simulink model "SDS_CBC_forcopyandpaste"  (R2018b)
settings: Solver=VariableStepAuto  StartTime=0.0  StopTime=10.0  RelTol=1e-3
PostLoadFcn:
  | , if any(exist('dsrtsu_mdlpostloadfcn', 'file') == [2, 3, 6]), try dsrtsu_mdlpostloadfcn('Execute', bdroot); catch fprintf('Error in PostLoadFcn (dsrtsu_mdlpostloadfcn) for model "%s":\n %s\n', bdroot, lasterr); end, end,
libraries: rtican x2, simulink x1
settings Model: DSRTSU_INTERNAL_RTI_VER=520  DSRTSU_INTERNAL_RTI_TYPE=rti1401  Creator=cordunoalbarran  LastModifiedBy=cordunoalbarran

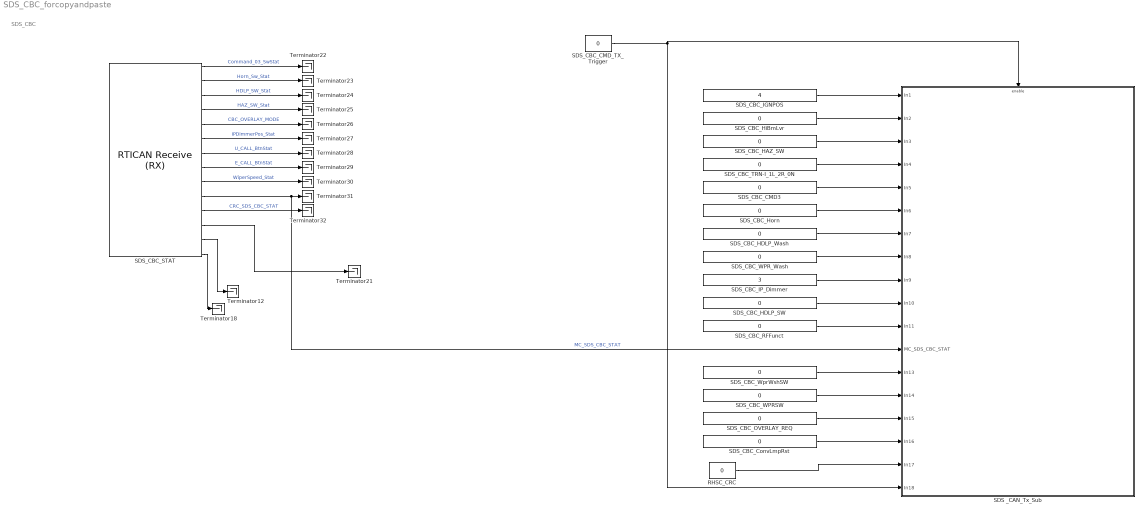
== system SDS_CBC_forcopyandpaste ==
  note: SDS_CBC
  RHSC_CRC : Constant  Value=0  OutDataTypeStr=Inherit: Inherit via back propagation
  "SDS _CAN_Tx_Sub " : Subsystem
  SDS_CBC_CMD3 : Constant  Value=0
  SDS_CBC_CMD_TX_Trigger : Constant  Value=0  OutDataTypeStr=Inherit: Inherit via back propagation
  SDS_CBC_ConvLmpRst : Constant  Value=0
  SDS_CBC_HAZ_SW : Constant  Value=0
  SDS_CBC_HDLP_SW : Constant  Value=0
  SDS_CBC_HDLP_Wash : Constant  Value=0
  SDS_CBC_HiBmLvr : Constant  Value=0
  SDS_CBC_Horn : Constant  Value=0
  SDS_CBC_IGNPOS : Constant  Value=4  OutMin=0  OutMax=6
  SDS_CBC_IP_Dimmer : Constant  Value=3
  SDS_CBC_OVERLAY_REQ : Constant  Value=0
  SDS_CBC_RFFunct : Constant  Value=0
  SDS_CBC_STAT : rtican/RTICAN Receive (RX)   Reserved1=[]  Reserved2=[]  Reserved3=[]  Reserved4=[]  SfcnMessage=[]  Msg_Struct=[]  BoardTypeNo=[]  BoardNo=[]  ChannelNo=[]  Parameters=[]  DialogFcn=[]  UnitName=[]  Revision=[]  UnitValues=[]  DSProperties=struct('RTI',struct('Version',uint32(5),'BlockType',struct('isSLSource',uint8(1),'isSLSink',uint8(1),'isHWSource',uint8(0),'isHWSink',uint8(0),'isSetup',uint8(0),'isInline',uint8(1),'isNonInline',uint8(0),'isInterrupt',uint8(0),'isChannelwise',uint8(0)),'IOBoardType','RTICAN','UnitType','MESSAGE','Identifier','RX','DialogType','MSVC','BlockSet','RTICAN','SlaveProcessor','CAN'))  RTIBlockInterface=struct('OutputPortsWidth',int32([1 1 1 1 1 1 1 1 1 1 1 1 1 1]),'OutputPortsActive',ones(1,14),'OutputPortsName',{{'Command_03_SwStat','Horn_Sw_Stat','HDLP_SW_Stat','HAZ_SW_Stat','CBC_OVERLAY_MODE','IPDimmerPos_Stat','U_CALL_BtnStat','E_CALL_BtnStat','WiperSpeed_Stat','MC_SDS_CBC_STAT','CRC_SDS_CBC_STAT',['RX status'],['RX time'],['RX delta time']}},'OutputPortsDataType',{{'SS_UINT8','SS_BOOLEAN','SS_UINT8','SS_BOOLEAN','SS_UINT8','SS_UINT8','SS_UINT8','SS_UINT8','SS_UINT8','SS_UINT8','SS_UINT8','SS_DOUBLE','SS_DOUBLE','SS_DOUBLE'}},'OutputPortsLabel',{{'Command_03_SwStat','Horn_Sw_Stat','HDLP_SW_Stat','HAZ_SW_Stat','CBC_OVERLAY_MODE','IPDimmerPos_Stat','U_CALL_BtnStat','E_CALL_BtnStat','WiperSpeed_Stat','MC_SDS_CBC_STAT','CRC_SDS_CBC_STAT','','',''}},'OutputPortsLabelMode','ON','InputPortsWidth',int32(0),'InputPortsActive',0,'DialogFcn','rtican_message_interface_gui','BlockDisplay',{{'','center'}},'IconTransparency','on','ParameterTunableNames',{{}},'InitLevel',3,'BlockName',struct('Token',{{'SDS_CBC_STAT'}}),'SampleTime',{{-1}},'TriggerPort',{{'none'}},'EnablePort',{{'none'}})  RTIBlockParameters=struct('BoardTypeNo',{{1,'OFF',[]}},'BoardNo',{{1,'ON',[1 16]}},'ChannelNo',{{1,'ON',[1 2]}},'Parameters',{{struct('DataFileSupport',struct('DataFileSelectedMaster',1,'DataFileSelectedLocal',1,'DataFileName',['c:\intrepidcs\pacifica dbc\e4a_r4_ccan_cr11690_mod.dbc|'],'DataFileDate',{{{['26-Feb-2019 09:25:05']}}},'SelectedFile',['..\..\..\..\..\..\..\intrepidcs\pacifica dbc\e4a_r4_ccan_cr11690_mod.dbc'],'InterfaceFcn','rtican_dbc_file_parser'),'Options',struct('StatusSelected',1,'TimeSelected',1,'DeltaTimeSelected',1,'BytePortSelected',0,'MessageLengthSelected',0,'TriggerPort',struct('Selected',0,'TriggerType',0),'UserCoding',struct('Selected',0,'InterfaceFile','UserDecodingFile','FcnName','UserDecodeFcn','InportSelected',0,'InportWidth',1,'OutportSelected',0,'OutportWidth',1),'EnablePortSelected',0,'SignalOnPortnameSelected',1,'UseRXService',0),'Message',struct('MsgOnBlocknameSelected',1,'MsgName','SDS_CBC_STAT','MsgIdFormat',0,'MsgId',858,'MsgLength',5,'NumSignals',11,'SampleTime',-1,'Signal',struct('SgnName',{'Command_03_SwStat','Horn_Sw_Stat','HDLP_SW_Stat','HAZ_SW_Stat','CBC_OVERLAY_MODE','IPDimmerPos_Stat','U_CALL_BtnStat','E_CALL_BtnStat','WiperSpeed_Stat','MC_SDS_CBC_STAT','CRC_SDS_CBC_STAT'},'SgnStartBit',{0,2,4,7,13,16,20,22,24,28,32},'SgnLength',{2,1,3,1,3,4,2,2,2,4,8},'SgnType',{0,0,0,0,0,0,0,0,0,0,0},'ModeValue',{-1,-1,-1,-1,-1,-1,-1,-1,-1,-1,-1},'DataType',{0,0,0,0,0,0,0,0,0,0,0},'ByteLayout',{0,0,0,0,0,0,0,0,0,0,0},'Factor',{1,1,1,1,1,1,1,1,1,1,1},'Offset',{0,0,0,0,0,0,0,0,0,0,0},'SgnComment',{{['Steering wheel switch 3 - Actual Switch Status (mode button)']},{['Physical Horn Pad Status']},{['Headlamp switch actual status']},{['Hazard Switch Actual Status; Not Pressed = [0], Pressed = [1];']},{['CBC Overlay Mode']},{['IP Dimmer Position Status to RHSC2']},{['Ucall button status to RHSC2']},{['Ecall button status to RHSC2']},{['Speed of wiper from RLS']},{['Message counter']},{['CRC-checksum byte 1 to 4 according to SAE J1850']}},'SgnUnit',{'','','','','','','','','','',''},'Min',{0,0,0,0,0,0,0,0,0,0,0},'Max',{0,0,0,0,0,0,0,0,0,15,0},'SLDataType',{'SS_UINT8','SS_BOOLEAN','SS_UINT8','SS_BOOLEAN','SS_UINT8','SS_UINT8','SS_UINT8','SS_UINT8','SS_UINT8','SS_UINT8','SS_UINT8'}),'MsgIdNumFormat',0,'MsgComment',{{''}}),'Version',1.2,'general',struct('isFromLib',0)),'OFF',[]}},'GroupId',{{struct('Group',{{'RTICAN'}},'No',1,'Behavior',{{'NAMECHANGE'}},'BlockType',{{'SINK'}},'NameChangeFlag',0),'OFF',[]}},'SFcnRTICANMessage',{{struct('MsgType','RX','SFcnPortType','Scalar','MsgName','SDS_CBC_STAT','MsgIdFormat','STD','MsgId',858,'MsgLength',5,'NumSignals',11,'SampleTime',-1,'Signal',struct('SgnName',{'Command_03_SwStat','Horn_Sw_Stat','HDLP_SW_Stat','HAZ_SW_Stat','CBC_OVERLAY_MODE','IPDimmerPos_Stat','U_CALL_BtnStat','E_CALL_BtnStat','WiperSpeed_Stat','MC_SDS_CBC_STAT','CRC_SDS_CBC_STAT'},'SgnStartBit',{0,2,4,7,13,16,20,22,24,28,32},'SgnLength',{2,1,3,1,3,4,2,2,2,4,8},'SgnType',{'standard','standard','standard','standard','standard','standard','standard','standard','standard','standard','standard'},'ModeValue',{-1,-1,-1,-1,-1,-1,-1,-1,-1,-1,-1},'DataType',{['unsigned int'],['unsigned int'],['unsigned int'],['unsigned int'],['unsigned int'],['unsigned int'],['unsigned int'],['unsigned int'],['unsigned int'],['unsigned int'],['unsigned int']},'ByteLayout',{['little endian'],['little endian'],['little endian'],['little endian'],['little endian'],['little endian'],['little endian'],['little endian'],['little endian'],['little endian'],['little endian']},'Factor',{1,1,1,1,1,1,1,1,1,1,1},'Offset',{0,0,0,0,0,0,0,0,0,0,0},'SLDataType',{'SS_UINT8','SS_BOOLEAN','SS_UINT8','SS_BOOLEAN','SS_UINT8','SS_UINT8','SS_UINT8','SS_UINT8','SS_UINT8','SS_UINT8','SS_UINT8'}),'StatusSelected','yes','TimeSelected','yes','DeltaTimeSelected','yes','BytePortSelected','no','MessageLengthSelected','no','TriggerPort',struct('Selected','no','TriggerType',0),'UserCoding',struct('Selected','no','InterfaceFile','UserDecodingFile','FcnName','UserDecodeFcn','InportSelected','no','InportWidth',1,'OutportSelected','no','OutportWidth',1),'EnablePortSelected','no','UseRXService','no','BoardType','DS1','BoardNo',1,'ControllerNo',1),'OFF',[]}},'TLCFileName',{{'rtican_rx_message','OFF',[]}})  RTISFcnParameters=struct('SFcnRTICANMessage','struct','TLCFileName','char')  RTIBlockParaDefault=struct('BoardTypeNo',4302,'BoardNo',1,'ChannelNo',1,'Parameters',struct('DataFileSupport',struct('DataFileSelectedMaster',0,'DataFileSelectedLocal',0,'DataFileName','','DataFileDate','','SelectedFile',['<no file selected>']),'Options',struct('StatusSelected',1,'TimeSelected',1,'DeltaTimeSelected',1,'BytePortSelected',0,'MessageLengthSelected',0,'TriggerPort',struct('Selected',0,'TriggerType','rising'),'UserCoding',struct('Selected',0,'InterfaceFile','UserDecodingFile','FcnName','UserDecodeFcn','InportSelected',0,'InportWidth',1,'OutportSelected',0,'OutportWidth',1),'EnablePortSelected',0,'SignalOnPortnameSelected',1,'UseRXService',0),'Message',struct('MsgOnBlocknameSelected',0,'MsgName',['RX Message'],'MsgIdFormat',0,'MsgId',100,'MsgLength',8,'NumSignals',1,'SampleTime',-1,'Signal',struct('SgnName',['RX signal'],'SgnStartBit',0,'SgnLength',8,'SgnType',0,'ModeValue',-1,'DataType',0,'SLDataType','SS_DOUBLE','ByteLayout',0,'Factor',1,'Offset',0,'Min',0,'Max',255,'SgnComment',{{}},'SgnUnit',''),'MsgIdNumFormat',0,'MsgComment',{{''}}),'Version',1.2,'general',struct('isFromLib',1)),'GroupId',struct('Group',{{'RTICAN'}},'No',1,'Behavior',{{'NAMECHANGE'}},'BlockType',{{'SINK'}},'NameChangeFlag',0),'SFcnRTICANMessage',struct('MsgType','RX','MsgName',['RX Message'],'MsgIdFormat','STD','MsgId',100,'MsgLength',8,'NumSignals',1,'SampleTime',-1,'Signal',struct('SgnName',['RX signal'],'SgnStartBit',0,'SgnLength',8,'SgnType','standard','ModeValue',-1,'DataType',['unsigned int'],'ByteLayout',['little endian'],'SLDataType','SS_DOUBLE','Factor',1,'Offset',0),'StatusSelected','yes','TimeSelected','yes','DeltaTimeSelected','yes','BytePortSelected','no','MessageLengthSelected','no','EnablePortSelected','no','UserCoding',struct('Selected','no','InterfaceFile','UserDecodingFile','FcnName','UserDecodeFcn','InportSelected','no','InportWidth',1,'OutportSelected','no','OutportWidth',1),'TriggerPort',struct('Selected','no','TriggerType','rising'),'UseRXService','no','BoardType','DS4302','BoardNo',1,'ControllerNo',1,'SFcnPortType','Scalar'),'TLCFileName','rtican_rx_message')
      settings: AttributesFormatString=Group Id: RTICAN1\n  SourceProductName=dSPACE RTI CAN Blockset
  SDS_CBC_TRN-I_1L_2R_0N : Constant  Value=0
  SDS_CBC_WPRSW : Constant  Value=0
  SDS_CBC_WPR_Wash : Constant  Value=0
  SDS_CBC_WprWshSW : Constant  Value=0
  Terminator{12,18,21..32} (14 alike) : Terminator
  wires:
  SDS_CBC_OVERLAY_REQ/1 -> "SDS _CAN_Tx_Sub "/15(In15)
  SDS_CBC_WPR_Wash/1 -> "SDS _CAN_Tx_Sub "/8(In8)
  SDS_CBC_ConvLmpRst/1 -> "SDS _CAN_Tx_Sub "/16(In16)
  SDS_CBC_IP_Dimmer/1 -> "SDS _CAN_Tx_Sub "/9(In9)
  SDS_CBC_RFFunct/1 -> "SDS _CAN_Tx_Sub "/11(In11)
  RHSC_CRC/1 -> "SDS _CAN_Tx_Sub "/17(In17)
  SDS_CBC_HDLP_SW/1 -> "SDS _CAN_Tx_Sub "/10(In10)
  SDS_CBC_STAT/9 -> Terminator30/1  "WiperSpeed_Stat"
  SDS_CBC_STAT/4 -> Terminator25/1  "HAZ_SW_Stat"
  SDS_CBC_Horn/1 -> "SDS _CAN_Tx_Sub "/6(In6)
  SDS_CBC_STAT/3 -> Terminator24/1  "HDLP_SW_Stat"
  SDS_CBC_TRN-I_1L_2R_0N/1 -> "SDS _CAN_Tx_Sub "/4(In4)
  SDS_CBC_CMD3/1 -> "SDS _CAN_Tx_Sub "/5(In5)
  SDS_CBC_STAT/10 -> Terminator31/1, "SDS _CAN_Tx_Sub "/12(MC_SDS_CBC_STAT)  "MC_SDS_CBC_STAT"
  SDS_CBC_WPRSW/1 -> "SDS _CAN_Tx_Sub "/14(In14)
  SDS_CBC_HDLP_Wash/1 -> "SDS _CAN_Tx_Sub "/7(In7)
  SDS_CBC_HAZ_SW/1 -> "SDS _CAN_Tx_Sub "/3(In3)
  SDS_CBC_STAT/7 -> Terminator28/1  "U_CALL_BtnStat"
  SDS_CBC_STAT/5 -> Terminator26/1  "CBC_OVERLAY_MODE"
  SDS_CBC_STAT/14 -> Terminator18/1
  SDS_CBC_HiBmLvr/1 -> "SDS _CAN_Tx_Sub "/2(In2)
  SDS_CBC_STAT/6 -> Terminator27/1  "IPDimmerPos_Stat"
  SDS_CBC_STAT/2 -> Terminator23/1  "Horn_Sw_Stat"
  SDS_CBC_STAT/11 -> Terminator32/1  "CRC_SDS_CBC_STAT"
  SDS_CBC_STAT/8 -> Terminator29/1  "E_CALL_BtnStat"
  SDS_CBC_IGNPOS/1 -> "SDS _CAN_Tx_Sub "/1(In1)
  SDS_CBC_WprWshSW/1 -> "SDS _CAN_Tx_Sub "/13(In13)
  SDS_CBC_STAT/12 -> Terminator21/1
  SDS_CBC_CMD_TX_Trigger/1 -> "SDS _CAN_Tx_Sub "/18(In18), "SDS _CAN_Tx_Sub "/Enable
  SDS_CBC_STAT/1 -> Terminator22/1  "Command_03_SwStat"
  SDS_CBC_STAT/13 -> Terminator12/1

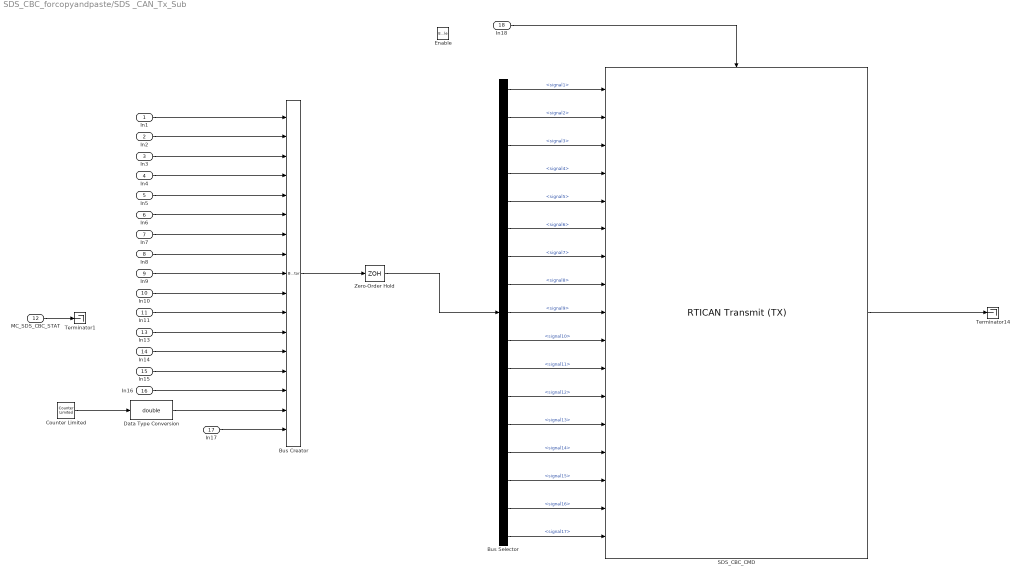
== system SDS_CBC_forcopyandpaste/SDS _CAN_Tx_Sub  ==
  In1 : Inport
  In2 : Inport  Port=2
  In3 : Inport  Port=3
  In4 : Inport  Port=4
  In5 : Inport  Port=5
  In6 : Inport  Port=6
  In7 : Inport  Port=7
  In8 : Inport  Port=8
  In9 : Inport  Port=9
  In10 : Inport  Port=10
  In11 : Inport  Port=11
  MC_SDS_CBC_STAT : Inport  Port=12
  In13 : Inport  Port=13
  In14 : Inport  Port=14
  In15 : Inport  Port=15
  In16 : Inport  Port=16
  In17 : Inport  Port=17
  In18 : Inport  Port=18
  Enable : EnablePort
  Bus Creator : BusCreator  Inputs=17
  Bus Selector : BusSelector  OutputSignals=signal1,signal2,signal3,signal4,signal5,signal6,signal7,signal8,signal9,signal10,signal11,signal12,signal13,signal14,signal15,signal16,signal17
  Counter Limited : simulink/Sources/Counter Limited  uplimit=15  tsamp=0.1
  Data Type Conversion : DataTypeConversion  OutDataTypeStr=double
  SDS_CBC_CMD : rtican/RTICAN Transmit (TX)   Reserved1=[]  Reserved2=[]  Reserved3=[]  Reserved4=[]  SfcnMessage=[]  Msg_Struct=[]  BoardTypeNo=[]  BoardNo=[]  ChannelNo=[]  Parameters=[]  DialogFcn=[]  UnitName=[]  Revision=[]  UnitValues=[]  DSProperties=struct('RTI',struct('Version',uint32(5),'BlockType',struct('isSLSource',uint8(1),'isSLSink',uint8(1),'isHWSource',uint8(0),'isHWSink',uint8(0),'isSetup',uint8(0),'isInline',uint8(1),'isNonInline',uint8(0),'isInterrupt',uint8(0),'isChannelwise',uint8(0)),'IOBoardType','RTICAN','UnitType','MESSAGE','Identifier','TX','DialogType','MSVC','BlockSet','RTICAN','SlaveProcessor','CAN'))  RTIBlockInterface=struct('InputPortsWidth',int32([1 1 1 1 1 1 1 1 1 1 1 1 1 1 1 1 1]),'InputPortsActive',ones(1,17),'InputPortsName',{{'IgnPos_Cmd','HiBmLvr_Cmd','HAZ_SW_Cmd','TurnIndLvr_Cmd','Command_03_Cmd','Horn_Sw_Cmd','HDLP_Wash_Cmd','WprWash_R_Sw_Posn_V3_Cmd','IPDimmerPos_Cmd','HDLP_Sw_Cmd','RFFuncReq_Cmd','WprWashSw_Psd_Cmd','WprSw6Posn_Cmd','SDS_CBC_OverlayReq','ConvLmpRst_Cmd','MC_SDS_CBC_CMD','CRC_SDS_CBC_CMD'}},'InputPortsDataType',{{'SS_UINT8','SS_UINT8','SS_BOOLEAN','SS_UINT8','SS_UINT8','SS_BOOLEAN','SS_BOOLEAN','SS_UINT8','SS_UINT8','SS_UINT8','SS_UINT8','SS_UINT8','SS_UINT8','SS_UINT8','SS_BOOLEAN','SS_UINT8','SS_UINT8'}},'OutputPortsWidth',int32(1),'OutputPortsActive',1,'OutputPortsName',{{['TX status']}},'DialogFcn','rtican_message_interface_gui','BlockDisplay',{{'','center'}},'IconTransparency','on','InitLevel',3,'BlockName',struct('Token',{{'SDS_CBC_CMD'}}),'SampleTime',{{-1}},'TriggerPort',{{'none'}},'EnablePort',{{'yes'}})  RTIBlockParameters=struct('BoardTypeNo',{{1,'OFF',[]}},'BoardNo',{{1,'ON',[1 16]}},'ChannelNo',{{1,'ON',[1 2]}},'Parameters',{{struct('DataFileSupport',struct('DataFileSelectedMaster',1,'DataFileSelectedLocal',1,'DataFileName',['c:\intrepidcs\pacifica dbc\e4a_r4_ccan_cr11690_mod.dbc|'],'DataFileDate',{{{['26-Feb-2019 09:25:05']}}},'SelectedFile',['..\..\..\..\..\..\..\intrepidcs\pacifica dbc\e4a_r4_ccan_cr11690_mod.dbc']),'Options',struct('StatusSelected',1,'TimeSelected',0,'DeltaTimeSelected',0,'DelayTimeSelected',0,'DelayTimeTXCommandSelected',0,'EncodeSetUnusedBitsToOne',0,'EnableMsgLoopback',0,'TriggerPort',struct('Selected',0,'TriggerType',0),'EnablePortSelected',1,'SignalOnPortnameSelected',1,'UserCoding',struct('Selected',1,'InterfaceFile','UserEncodingFile','FcnName','Message_CRC_Encoder','InportSelected',0,'InportWidth',1,'OutportSelected',0,'OutportWidth',1),'TerminationMsg',struct('Selected',0,'Byte0_7','0'),'InitialMsg',struct('Selected',0,'Byte0_7','0')),'Message',struct('MsgOnBlocknameSelected',1,'MsgName','SDS_CBC_CMD','MsgIdFormat',0,'MsgId',857,'MsgLength',8,'NumSignals',17,'SampleTime',-1,'StartTime',struct('Selected',1,'Value',0),'AutoRepeatTime',struct('Selected',1,'Value',0.1),'Timeout',struct('Selected',0,'Value',0.1),'DelayTime',struct('Selected',0,'Value',0.1),'Signal',struct('SgnName',{'IgnPos_Cmd','HiBmLvr_Cmd','HAZ_SW_Cmd','TurnIndLvr_Cmd','Command_03_Cmd','Horn_Sw_Cmd','HDLP_Wash_Cmd','WprWash_R_Sw_Posn_V3_Cmd','IPDimmerPos_Cmd','HDLP_Sw_Cmd','RFFuncReq_Cmd','WprWashSw_Psd_Cmd','WprSw6Posn_Cmd','SDS_CBC_OverlayReq','ConvLmpRst_Cmd','MC_SDS_CBC_CMD','CRC_SDS_CBC_CMD'},'SgnStartBit',{0,3,5,6,8,12,13,14,20,32,35,42,44,48,51,52,56},'SgnLength',{3,2,1,2,2,1,1,2,4,3,5,2,4,3,1,4,8},'SgnType',{0,0,0,0,0,0,0,0,0,0,0,0,0,0,0,0,0},'ModeValue',{-1,-1,-1,-1,-1,-1,-1,-1,-1,-1,-1,-1,-1,-1,-1,-1,-1},'DataType',{0,0,0,0,0,0,0,0,0,0,0,0,0,0,0,0,0},'ByteLayout',{0,0,0,0,0,0,0,0,0,0,0,0,0,0,0,0,0},'Factor',{1,1,1,1,1,1,1,1,1,1,1,1,1,1,1,1,1},'Offset',{0,0,0,0,0,0,0,0,0,0,0,0,0,0,0,0,0},'SgnComment',{{['Driver requested ignition position - Overlay from SDS']},{['High beam lever state - Overlay from SDS']},{['Hazard Switch Command; Not Pressed = [0]; Pressed = [1];']},{['Turn indicator lever state - Overlay from SDS']},{['Steering wheel switch 3 (mode button) - Overlay from SDS']},{['Horn Activation Request from SDS, Off = [0], On = [1];']},{['Headlight washer pump control - Overlay from SDS, Off = [0], On = [1];']},{['Backlite wiper/washer switch position - Overlay from SDS']},{['IP Dimmer Position Cmd from RHSC2']},{['Headlamp Switch Command']},{['Basic request (RKE, PE, Remstart) - Overlay from SDS']},{['Front wiper switch pressed']},{['Wiper switch (6 stages) position - Overlay from SDS']},{['SDS CBC overlay request']},{['Convenience Lamp Reset Requeset, No Request = [0], Reset = [1]; ']},{['Message counter']},{['CRC-checksum byte 1 to 7 according to SAE J1850']}},'SgnUnit',{'','','','','','','','','','','','','','','','',''},'Min',{0,0,0,0,0,0,0,0,0,0,0,0,0,0,0,0,0},'Max',{0,0,0,0,0,0,0,0,0,0,0,0,0,0,0,15,255},'SLDataType',{'SS_UINT8','SS_UINT8','SS_BOOLEAN','SS_UINT8','SS_UINT8','SS_BOOLEAN','SS_BOOLEAN','SS_UINT8','SS_UINT8','SS_UINT8','SS_UINT8','SS_UINT8','SS_UINT8','SS_UINT8','SS_BOOLEAN','SS_UINT8','SS_UINT8'}),'MsgIdNumFormat',0,'MsgComment',{{''}}),'Version',1.2,'general',struct('isFromLib',0)),'OFF',[]}},'GroupId',{{struct('Group',{{'RTICAN'}},'No',1,'Behavior',{{'NAMECHANGE'}},'BlockType',{{'SINK'}},'NameChangeFlag',0),'OFF',[]}},'SFcnRTICANMessage',{{struct('MsgType','TX','SFcnPortType','Scalar','MsgName','SDS_CBC_CMD','MsgIdFormat','STD','MsgId',857,'MsgLength',8,'NumSignals',17,'SampleTime',-1,'StartTime',struct('Selected','yes','Value',0),'AutoRepeatTime',struct('Selected','yes','Value',0.1),'Timeout',struct('Selected','no','Value',0.1),'Signal',struct('SgnName',{'IgnPos_Cmd','HiBmLvr_Cmd','HAZ_SW_Cmd','TurnIndLvr_Cmd','Command_03_Cmd','Horn_Sw_Cmd','HDLP_Wash_Cmd','WprWash_R_Sw_Posn_V3_Cmd','IPDimmerPos_Cmd','HDLP_Sw_Cmd','RFFuncReq_Cmd','WprWashSw_Psd_Cmd','WprSw6Posn_Cmd','SDS_CBC_OverlayReq','ConvLmpRst_Cmd','MC_SDS_CBC_CMD','CRC_SDS_CBC_CMD'},'SgnStartBit',{0,3,5,6,8,12,13,14,20,32,35,42,44,48,51,52,56},'SgnLength',{3,2,1,2,2,1,1,2,4,3,5,2,4,3,1,4,8},'SgnType',{'standard','standard','standard','standard','standard','standard','standard','standard','standard','standard','standard','standard','standard','standard','standard','standard','standard'},'ModeValue',{-1,-1,-1,-1,-1,-1,-1,-1,-1,-1,-1,-1,-1,-1,-1,-1,-1},'DataType',{['unsigned int'],['unsigned int'],['unsigned int'],['unsigned int'],['unsigned int'],['unsigned int'],['unsigned int'],['unsigned int'],['unsigned int'],['unsigned int'],['unsigned int'],['unsigned int'],['unsigned int'],['unsigned int'],['unsigned int'],['unsigned int'],['unsigned int']},'ByteLayout',{['little endian'],['little endian'],['little endian'],['little endian'],['little endian'],['little endian'],['little endian'],['little endian'],['little endian'],['little endian'],['little endian'],['little endian'],['little endian'],['little endian'],['little endian'],['little endian'],['little endian']},'Factor',{1,1,1,1,1,1,1,1,1,1,1,1,1,1,1,1,1},'Offset',{0,0,0,0,0,0,0,0,0,0,0,0,0,0,0,0,0},'SLDataType',{'SS_UINT8','SS_UINT8','SS_BOOLEAN','SS_UINT8','SS_UINT8','SS_BOOLEAN','SS_BOOLEAN','SS_UINT8','SS_UINT8','SS_UINT8','SS_UINT8','SS_UINT8','SS_UINT8','SS_UINT8','SS_BOOLEAN','SS_UINT8','SS_UINT8'}),'StatusSelected','yes','TimeSelected','no','DeltaTimeSelected','no','DelayTimeSelected','no','DelayTimeTXCommandSelected','no','EncodeSetUnusedBitsToOne','no','EnableMsgLoopback','no','TriggerPort',struct('Selected','no','TriggerType',0),'EnablePortSelected','yes','UserCoding',struct('Selected','yes','InterfaceFile','UserEncodingFile','FcnName','Message_CRC_Encoder','InportSelected','no','InportWidth',1,'OutportSelected','no','OutportWidth',1),'TerminationMsg',struct('Selected','no','Byte0','0x00','Byte1','0x00','Byte2','0x00','Byte3','0x00','Byte4','0x00','Byte5','0x00','Byte6','0x00','Byte7','0x00'),'InitialMsg',struct('Selected','no','Byte0','0x00','Byte1','0x00','Byte2','0x00','Byte3','0x00','Byte4','0x00','Byte5','0x00','Byte6','0x00','Byte7','0x00'),'BoardType','DS1','BoardNo',1,'ControllerNo',1),'OFF',[]}},'TLCFileName',{{'rtican_tx_message','OFF',[]}})  RTISFcnParameters=struct('SFcnRTICANMessage','struct','TLCFileName','char')  RTIBlockParaDefault=struct('BoardTypeNo',4302,'BoardNo',1,'ChannelNo',1,'Parameters',struct('DataFileSupport',struct('DataFileSelectedMaster',0,'DataFileSelectedLocal',0,'DataFileName','','DataFileDate','','SelectedFile',['<no file selected>']),'Options',struct('StatusSelected',1,'TimeSelected',1,'DeltaTimeSelected',1,'DelayTimeSelected',1,'DelayTimeTXCommandSelected',0,'EncodeSetUnusedBitsToOne',0,'EnableMsgLoopback',0,'TriggerPort',struct('Selected',0,'TriggerType','rising'),'EnablePortSelected',0,'SignalOnPortnameSelected',1,'UserCoding',struct('Selected',0,'InterfaceFile','UserEncodingFile','FcnName','UserEncodeFcn','InportSelected',0,'InportWidth',1,'OutportSelected',0,'OutportWidth',1),'TerminationMsg',struct('Selected',0,'Byte0_7','0'),'InitialMsg',struct('Selected',0,'Byte0_7','0')),'Message',struct('MsgOnBlocknameSelected',0,'MsgName',['TX Message'],'MsgIdFormat',0,'MsgId',100,'MsgLength',8,'NumSignals',1,'SampleTime',-1,'StartTime',struct('Selected',0,'Value',0),'AutoRepeatTime',struct('Selected',0,'Value',0.1),'Timeout',struct('Selected',0,'Value',0.1),'DelayTime',struct('Selected',0,'Value',0.1),'Signal',struct('SgnName',['TX signal'],'SgnStartBit',0,'SgnLength',8,'SgnType',0,'ModeValue',-1,'DataType',0,'SLDataType','SS_DOUBLE','ByteLayout',0,'Factor',1,'Offset',0,'Min',0,'Max',255,'SgnComment',{{}},'SgnUnit',''),'MsgIdNumFormat',0,'MsgComment',{{''}}),'Version',1.2,'general',struct('isFromLib',1)),'GroupId',struct('Group',{{'RTICAN'}},'No',1,'Behavior',{{'NAMECHANGE'}},'BlockType',{{'SINK'}},'NameChangeFlag',0),'SFcnRTICANMessage',struct('MsgType','TX','MsgName',['TX Message'],'MsgIdFormat','STD','MsgId',100,'MsgLength',2,'NumSignals',1,'SampleTime',-1,'StartTime',struct('Selected','no','Value',0),'AutoRepeatTime',struct('Selected','no','Value',0.1),'Timeout',struct('Selected','no','Value',0.1),'DelayTime',struct('Selected','no','Value',0.1),'Signal',struct('SgnName',['TX signal'],'SgnStartBit',0,'SgnLength',8,'SgnType','standard','ModeValue',-1,'DataType',['unsigned int'],'ByteLayout',['little endian'],'SLDataType','SS_DOUBLE','Factor',1,'Offset',0),'StatusSelected','yes','TimeSelected','yes','DeltaTimeSelected','yes','DelayTimeSelected','yes','EnablePortSelected','no','EnableMsgLoopback','no','DelayTimeTXCommandSelected','no','EncodeSetUnusedBitsToOne','no','UserCoding',struct('Selected','no','InterfaceFile','UserDecodingFile','FcnName','UserDecodeFcn','InportSelected','no','InportWidth',1,'OutportSelected','no','OutportWidth',1),'TerminationMsg',struct('Selected','no','Byte0','0x00','Byte1','0x00','Byte2','0x00','Byte3','0x00','Byte4','0x00','Byte5','0x00','Byte6','0x00','Byte7','0x00'),'InitialMsg',struct('Selected','no','Byte0','0x00','Byte1','0x00','Byte2','0x00','Byte3','0x00','Byte4','0x00','Byte5','0x00','Byte6','0x00','Byte7','0x00'),'TriggerPort',struct('Selected','no','TriggerType','rising'),'BoardType','DS4302','BoardNo',1,'ControllerNo',1,'SFcnPortType','Scalar'),'TLCFileName','rtican_tx_message')
      settings: AttributesFormatString=Group Id: RTICAN1\n  SourceProductName=dSPACE RTI CAN Blockset
  Terminator1 : Terminator
  Terminator14 : Terminator
  Zero-Order Hold : ZeroOrderHold  SampleTime=-1
  wires:
  SDS_CBC_CMD/1 -> Terminator14/1
  In18/1 -> SDS_CBC_CMD/Enable
  In1/1 -> Bus Creator/1
  In2/1 -> Bus Creator/2
  In3/1 -> Bus Creator/3
  In4/1 -> Bus Creator/4
  In5/1 -> Bus Creator/5
  In6/1 -> Bus Creator/6
  In7/1 -> Bus Creator/7
  In8/1 -> Bus Creator/8
  In9/1 -> Bus Creator/9
  In10/1 -> Bus Creator/10
  In11/1 -> Bus Creator/11
  In17/1 -> Bus Creator/17
  In13/1 -> Bus Creator/12
  In14/1 -> Bus Creator/13
  In15/1 -> Bus Creator/14
  In16/1 -> Bus Creator/15
  MC_SDS_CBC_STAT/1 -> Terminator1/1
  Bus Creator/1 -> Zero-Order Hold/1
  Zero-Order Hold/1 -> Bus Selector/1
  Bus Selector/1 -> SDS_CBC_CMD/1  "<signal1>"
  Bus Selector/2 -> SDS_CBC_CMD/2  "<signal2>"
  Bus Selector/3 -> SDS_CBC_CMD/3  "<signal3>"
  Bus Selector/4 -> SDS_CBC_CMD/4  "<signal4>"
  Bus Selector/5 -> SDS_CBC_CMD/5  "<signal5>"
  Bus Selector/6 -> SDS_CBC_CMD/6  "<signal6>"
  Bus Selector/7 -> SDS_CBC_CMD/7  "<signal7>"
  Bus Selector/8 -> SDS_CBC_CMD/8  "<signal8>"
  Bus Selector/9 -> SDS_CBC_CMD/9  "<signal9>"
  Bus Selector/10 -> SDS_CBC_CMD/10  "<signal10>"
  Bus Selector/11 -> SDS_CBC_CMD/11  "<signal11>"
  Bus Selector/12 -> SDS_CBC_CMD/12  "<signal12>"
  Bus Selector/13 -> SDS_CBC_CMD/13  "<signal13>"
  Bus Selector/14 -> SDS_CBC_CMD/14  "<signal14>"
  Bus Selector/15 -> SDS_CBC_CMD/15  "<signal15>"
  Bus Selector/16 -> SDS_CBC_CMD/16  "<signal16>"
  Bus Selector/17 -> SDS_CBC_CMD/17  "<signal17>"
  Counter Limited/1 -> Data Type Conversion/1
  Data Type Conversion/1 -> Bus Creator/16
